simulink model "cruise_control_2024"  (R2024b)
settings: Solver=ode5  StartTime=0.0  StopTime=10  FixedStep=0.01  RelTol=1e-3
values from neighbouring files (symbols this model uses):
  K = 0.0512797808763    [cruise_control_test.mat]
  Tau = 61.5357370516    [cruise_control_test.mat]
settings Model: Creator=Asus  LastModifiedBy=Asus
settings OptimizationCC: ZeroExternalMemoryAtStartup=off  ZeroInternalMemoryAtStartup=off
settings SFSimCC: SimCustomHeaderCode="extern \"C\" void compute_pid_gains(double m, double u0, double* Kp, double* Ki, double* Kd);"  SimUserSources=cruise_control.cpp  SimTargetLang=C++
settings RTWCC: CustomHeaderCode=controller.h  CustomSource=cruise_control.cpp  CustomInitializer=cruise_control.cpp  TargetLang=C++
settings GRTTargetCC: TargetLangStandard=C++11 (ISO)  CodeInterfacePackaging=C++ class

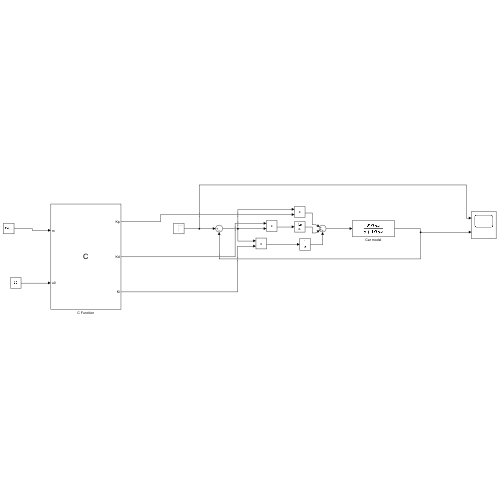
[thumbnail: Simulink's stored preview of the top-level diagram]
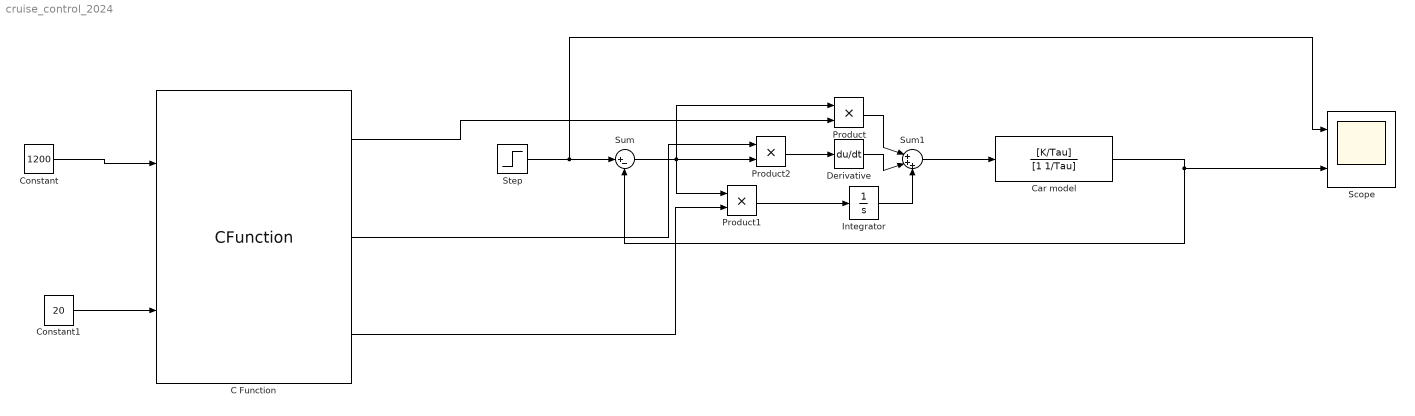
== system cruise_control_2024 ==
  C Function : CFunction  OutputCode=compute_pid_gains(m, u0, &Kp, &Ki, &Kd);  CodegenOutputCode=compute_pid_gains(m, u0, &Kp, &Ki, &Kd);  CustomCodeSettingLocation=ModelConfigurationParameters
  Car model : TransferFcn  Numerator=[K/Tau]  Denominator=[1 1/Tau]
  Constant : Constant  Value=1200
  Constant1 : Constant  Value=20
  Derivative : Derivative
  Integrator : Integrator
  Product : Product
  Product1 : Product
  Product2 : Product
  Scope : Scope  NumInputPorts=2
  Step : Step  After=60  SampleTime=0
  Sum : Sum  Inputs=|+-
  Sum1 : Sum  Inputs=|+++
  wires:
  Step/1 -> Scope/1, Sum/1
  Car model/1 -> Sum/2, Scope/2
  Constant/1 -> C Function/1
  Constant1/1 -> C Function/2
  Derivative/1 -> Sum1/2
  Product2/1 -> Derivative/1
  Product1/1 -> Integrator/1
  Sum1/1 -> Car model/1
  Integrator/1 -> Sum1/3
  Sum/1 -> Product2/2, Product1/1, Product/1
  C Function/1 -> Product/2
  Product/1 -> Sum1/1
  C Function/3 -> Product1/2
  C Function/2 -> Product2/1
